simulink model "M4_Control"  (R2026a)
settings: Solver=FixedStepDiscrete  FixedStep=0.1
PreLoadFcn:
  | createM4BusObjects
libraries: mpclib x1
settings Model: Creator=jeevan  LastModifiedBy=jeevan

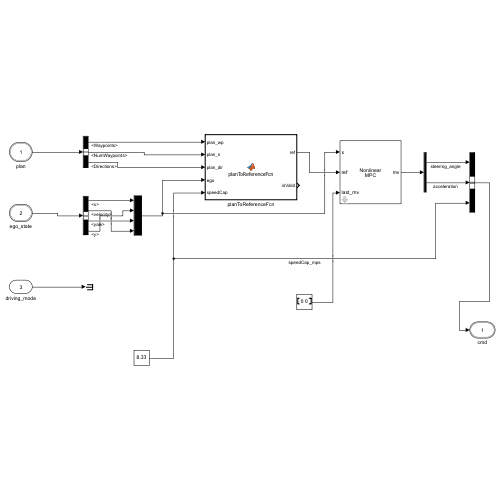
[thumbnail: Simulink's stored preview of the top-level diagram]
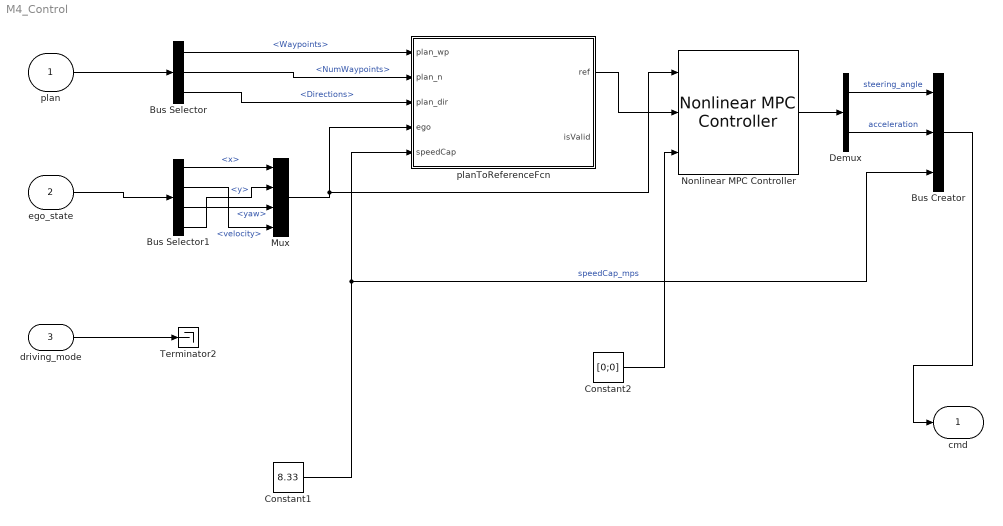
== system M4_Control ==
  plan : Inport  OutDataTypeStr=Bus: SihPlanBus  BusOutputAsStruct=on
  ego_state : Inport  Port=2  OutDataTypeStr=Bus: SihEgoBus  BusOutputAsStruct=on
  driving_mode : Inport  Port=3  OutDataTypeStr=Enum: DrivingMode  BusOutputAsStruct=on
  Bus Creator : BusCreator  Inputs=3  OutDataTypeStr=Bus: SihControlCmdBus
  Bus Selector : BusSelector  OutputSignals=Waypoints,NumWaypoints,Directions
  Bus Selector1 : BusSelector  OutputSignals=x,velocity,yaw,y
  Constant1 : Constant  Value=8.33
  Constant2 : Constant  Value=[0;0]
  Demux : Demux  Outputs=2
  Mux : Mux
  Nonlinear MPC Controller : mpclib/Nonlinear MPC Controller  nlmpcobj=nlobj  md_enabled=off  mvtarget_enabled=off  param_enabled=off  cost_enabled=off  mvseq_enabled=off  stateseq_enabled=off  ovseq_enabled=off  slack_enabled=off  status_enabled=off  ov_min=off  ov_max=off  mv_min=off  mv_max=off  mvrate_min=off  mvrate_max=off  state_min=off  state_max=off  ov_weight=off  mv_weight=off  mvrate_weight=off  ecr_weight=off  nlp_initialize=off  BlockDataType=double  UseObjectTs=on  UseMEX=off
  Terminator2 : Terminator
  planToReferenceFcn : MATLAB Function  TreatAsAtomicUnit=on
  cmd : Outport  OutDataTypeStr=Bus: SihControlCmdBus  BusOutputAsStruct=on
  wires:
  plan/1 -> Bus Selector/1
  ego_state/1 -> Bus Selector1/1
  driving_mode/1 -> Terminator2/1
  Bus Selector/1 -> planToReferenceFcn/1(plan_wp)  "<Waypoints>"
  Bus Selector/2 -> planToReferenceFcn/2(plan_n)  "<NumWaypoints>"
  Bus Selector/3 -> planToReferenceFcn/3(plan_dir)  "<Directions>"
  Mux/1 -> Nonlinear MPC Controller/1, planToReferenceFcn/4(ego)
  Constant1/1 -> planToReferenceFcn/5(speedCap), Bus Creator/3  "speedCap_mps"
  planToReferenceFcn/1(ref) -> Nonlinear MPC Controller/2
  Nonlinear MPC Controller/1 -> Demux/1
  Constant2/1 -> Nonlinear MPC Controller/3
  Demux/1 -> Bus Creator/1  "steering_angle"
  Demux/2 -> Bus Creator/2  "acceleration"
  Bus Creator/1 -> cmd/1
  Bus Selector1/1 -> Mux/1  "<x>"
  Bus Selector1/3 -> Mux/3  "<yaw>"
  Bus Selector1/2 -> Mux/4  "<velocity>"
  Bus Selector1/4 -> Mux/2  "<y>"

== matlab function M4_Control/planToReferenceFcn ==
  data: plan_wp input; ref output; plan_n input; plan_dir input; ego input; speedCap input; isValid output
function [ref, isValid] = planToReferenceFcn(plan_wp, plan_n, plan_dir, ego, speedCap)
%#codegen
Ts = 0.1;
p  = 20;

coder.varsize('W',     [5000 4], [1 0]);
coder.varsize('D',     [5000 1], [1 0]);
coder.varsize('keep',  [5000 1], [1 0]);
coder.varsize('s',     [5000 1], [1 0]);
coder.varsize('th',    [5000 1], [1 0]);
coder.varsize('vProf', [5000 1], [1 0]);

ref     = zeros(p, 4);
isValid = false;

N = double(plan_n);
if N < 2, return; end

W = plan_wp(1:N, :);
D = double(plan_dir(1:N));

seg  = hypot(diff(W(:,1)), diff(W(:,2)));
keep = [true; seg > 1e-6];
W = W(keep, :);
D = D(keep);
n = size(W, 1);
if n < 2, return; end

s = [0; cumsum(hypot(diff(W(:,1)), diff(W(:,2))))];

d2      = (W(:,1)-ego(1)).^2 + (W(:,2)-ego(2)).^2;
[~, i0] = min(d2);

sCusp = s(end);
for k = i0:n-1
    if D(k+1) ~= D(k), sCusp = s(k); break; end
end

th    = unwrap(W(:,3));
vProf = sign(W(:,4)) .* min(abs(W(:,4)), abs(speedCap));

sk = s(i0);
for k = 1:p
    vk = interp1(s, vProf, sk, 'linear', 'extrap');
    sk = sk + abs(vk)*Ts;
    if sk >= sCusp - 1e-6, sk = sCusp; end
    if sk >= s(end) - 1e-6, sk = s(end); end
    ref(k,1) = interp1(s, W(:,1), sk);
    ref(k,2) = interp1(s, W(:,2), sk);
    ref(k,3) = interp1(s, th,     sk);
    ref(k,4) = interp1(s, vProf,  sk);
end

ref(:,3) = unwrap(ref(:,3));
ref(:,3) = ref(:,3) + round((ego(3)-ref(1,3))/(2*pi))*2*pi;
isValid  = true;
